simulink model "Controller"  (R2022b)
settings: Solver=FixedStepDiscrete  StartTime=0.0  StopTime=10.0  FixedStep=CONTROL_CONST.dt  RelTol=1e-3
values from neighbouring files (symbols this model uses):
  CONTROL_EXPORT = Simulink.Parameter(CONTROL_EXPORT_VALUE)    [controller_model_init.m]
  CONTROL_PARAM = Simulink.Parameter(CONTROL_PARAM_VALUE)    [controller_model_init.m]
undefined symbols (not defined in the file or in its folder): actuator_cmd, CONTROL_CONST, CONTROL_PARAM_VALUE, ControlMode, DiscIntNeverNeededParam, Discrete, Time, timestamp
libraries: simulink x10, FMT_Model_Lib x2, aerolibasang x1, ctrlSharedLib x1
(part 2 of 2)

== matlab function Controller/Lateral_Longitudinal_Control/Altitude_Control/Calc_Height_Rate_Setpoint/computeMaxSpeedFromDistance ==
  data: jerk input; max_speed output; accel input; braking_distance input; final_speed input
function max_speed = fcn(jerk, accel, braking_distance, final_speed)
    sqr = @(f) f * f;
    b = 4.0 * sqr(accel) / jerk;
    c = -2.0 * accel * braking_distance - sqr(final_speed);
    max_speed = 0.5 * (-b + sqrt(sqr(b) - 4.0 * c));
    
    % 不要减速超过最终速度，即使保守的加速度请求时间要求减速更多
    max_speed = max(max_speed, final_speed);
end
